simulink model "oneFingerFBSim"  (R2015b)
settings: Solver=VariableStepAuto  StartTime=0.0  StopTime=1  RelTol=1e-3
settings Model: Creator=Ricardo  LastModifiedBy=Ricardo

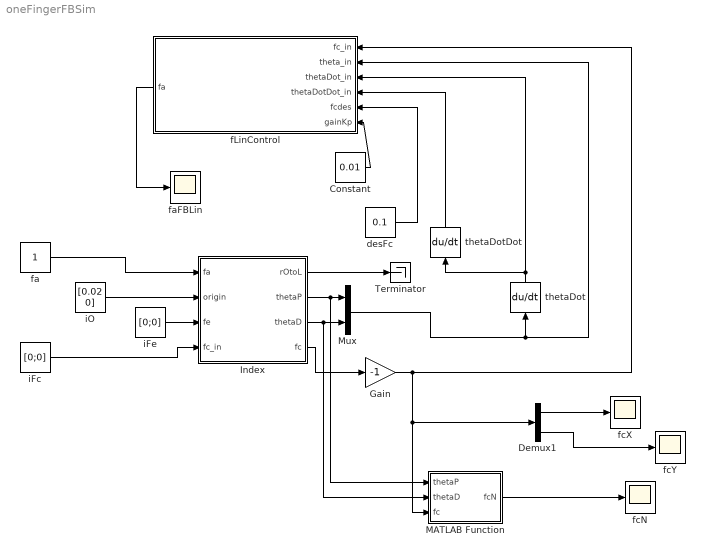
== system oneFingerFBSim ==
  Constant : Constant  Value=0.01
  Demux1 : Demux  Outputs=2
  Gain : Gain  Gain=-1
  Index : Subsystem
  MATLAB Function : MATLAB Function  TreatAsAtomicUnit=on
  Mux : Mux  Inputs=2
  Terminator : Terminator
  desFc : Constant  Value=0.1
  fLinControl : MATLAB Function  TreatAsAtomicUnit=on
  fa : Constant
  faFBLin : Scope
  fcN : Scope
  fcX : Scope
  fcY : Scope
  iFc : Constant  Value=[0;0]
  iFe : Constant  Value=[0;0]
  iO : Constant  Value=[0.02 0]
  thetaDot : Derivative
  thetaDotDot : Derivative
  wires:
  Demux1/1 -> fcX/1
  Demux1/2 -> fcY/1
  iO/1 -> Index/2(origin)
  Index/4(fc) -> Gain/1
  Index/2(thetaP) -> MATLAB Function/1(thetaP), Mux/1
  Index/3(thetaD) -> MATLAB Function/2(thetaD), Mux/2
  Mux/1 -> thetaDot/1, fLinControl/2(theta_in)
  desFc/1 -> fLinControl/5(fcdes)
  fLinControl/1(fa) -> faFBLin/1
  thetaDot/1 -> thetaDotDot/1, fLinControl/3(thetaDot_in)
  thetaDotDot/1 -> fLinControl/4(thetaDotDot_in)
  Constant/1 -> fLinControl/6(gainKp)
  iFe/1 -> Index/3(fe)
  Gain/1 -> MATLAB Function/3(fc), Demux1/1, fLinControl/1(fc_in)
  Index/1(rOtoL) -> Terminator/1
  MATLAB Function/1(fcN) -> fcN/1
  fa/1 -> Index/1(fa)
  iFc/1 -> Index/4(fc_in)

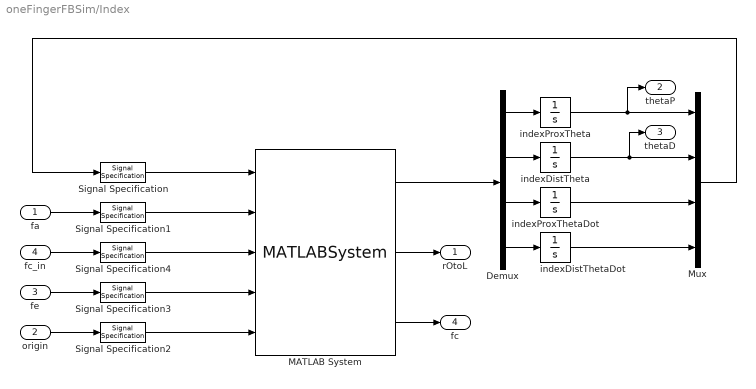
== system oneFingerFBSim/Index ==
  fa : Inport
  origin : Inport  Port=2
  fe : Inport  Port=3
  fc_in : Inport  Port=4
  Demux : Demux
  MATLAB System : MATLABSystem  System=Index  kP=-0.043  kD=-0.185  dP=-0.01  dD=-0.01  lP=0.1  lD=0.1  rP=0.02  rD=0.012  mP=0.02  mD=0.02  thetaP=pi/10  thetaD=pi/3  SimulateUsing=Interpreted execution
      mask Type: Index
      mask Display:
      | disp('Index');
      | port_label('input',1,'initVal');
      | port_label('input',2,'fa');
      | port_label('input',3,'fc');
      | port_label('input',4,'fe');
      | port_label('input',5,'origin');
      | port_label('output',1,'xDot');
      | port_label('output',2,'rOtoL');
      | port_label('output',3,'fc');
  Mux : Mux
  Signal Specification : SignalSpecification  Dimensions=4
  Signal Specification1 : SignalSpecification  Dimensions=1
  Signal Specification2 : SignalSpecification  Dimensions=2
  Signal Specification3 : SignalSpecification  Dimensions=2
  Signal Specification4 : SignalSpecification  Dimensions=2
  indexDistTheta : Integrator  InitialCondition=pi/3  ContinuousStateAttributes='indexDistTheta'
  indexDistThetaDot : Integrator  ContinuousStateAttributes='indexDistThetaDot'
  indexProxTheta : Integrator  InitialCondition=pi/10  ContinuousStateAttributes='indexProxTheta'
  indexProxThetaDot : Integrator  ContinuousStateAttributes='indexProxThetaDot'
  rOtoL : Outport
  thetaP : Outport  Port=2
  thetaD : Outport  Port=3
  fc : Outport  Port=4
  wires:
  Demux/1 -> indexProxTheta/1
  Demux/2 -> indexDistTheta/1
  Demux/3 -> indexProxThetaDot/1
  Demux/4 -> indexDistThetaDot/1
  MATLAB System/1 -> Demux/1
  indexProxTheta/1 -> Mux/1, thetaP/1
  indexDistTheta/1 -> Mux/2, thetaD/1
  indexProxThetaDot/1 -> Mux/3
  indexDistThetaDot/1 -> Mux/4
  Mux/1 -> Signal Specification/1
  Signal Specification/1 -> MATLAB System/1
  MATLAB System/2 -> rOtoL/1
  MATLAB System/3 -> fc/1
  Signal Specification1/1 -> MATLAB System/2
  fa/1 -> Signal Specification1/1
  origin/1 -> Signal Specification2/1
  Signal Specification2/1 -> MATLAB System/5
  fe/1 -> Signal Specification3/1
  Signal Specification3/1 -> MATLAB System/4
  fc_in/1 -> Signal Specification4/1
  Signal Specification4/1 -> MATLAB System/3

== matlab function oneFingerFBSim/MATLAB Function ==
  data: thetaP input; fcN output; thetaD input; fc input
function fcN = transFc(thetaP,thetaD,fc)
%#codegen

fcTN = [[cos(thetaP+thetaD),sin(thetaP+thetaD)];[-sin(thetaP+thetaD),cos(thetaP+thetaD)]]*fc;
fcN=fcTN(2,1);

== matlab function oneFingerFBSim/fLinControl ==
  data: fc_in input; theta_in input; fa output; thetaDot_in input; thetaDotDot_in input; fcdes input; gainKp input
function fa = fLinControl(fc_in,theta_in,thetaDot_in,thetaDotDot_in,fcdes,gainKp)
    theta = [theta_in(1);theta_in(2)];
    thetaDot = [thetaDot_in(1);thetaDot_in(2)];
    thetaDotDot = [thetaDotDot_in(1);thetaDotDot_in(2)];
	% Set model variables:
    kP = -0.043;
    kD = -0.185;
    dP = -0.01;
    dD = -0.01;
    lP = 0.1;
    lD = 0.1;
    rP = 0.02;
    rD = 0.012;
    aP = 0.1;
    aD = 0.1;
    mP = 0.02;
    mD = 0.02;
    theta0 = [pi/10;pi/3];
    IP = mP*(lP^2)/3;
    ID = mD*(lD^2)/12;
    % Set matrices
    K = [kP 0;
         0 kD];
    D = [dP 0;
         0 dD];
    Ja = [rP rD];
    Jc = [aP, 0;
          aD+lP*cos(theta(2,1)),aD]; 
    % Compute matrix parameters.
    alpha = IP + ID + (mP*(lP/2)^2) + mD*(lP^2+(lD/2)^2);
    beta = mD*lP*(lD/2);
    delta = ID+mD*(lD/2)^2;
    % Intertia matrix (M)
    M = [alpha+2*beta*cos(theta(2,1)) delta+beta*cos(theta(2,1));
         delta+beta*cos(theta(2,1)) delta];
    % Coriolis and Centrifugal matrix (C)
    C = [-beta*sin(theta(2,1))*thetaDot(2,1) ...
         -beta*sin(theta(2,1))*(thetaDot(1,1)+thetaDot(2,1));
         beta*sin(theta(2,1))*thetaDot(1,1) 0];
    springTau = K*(theta-theta0);
    damperTau = D*thetaDot;
    % Contact force
    fc = rotMat(theta(1,1)+theta(2,1))'*fc_in;
    fcN = fc(2,1);
    e = [0;fcdes-fcN];
    fa = pinv(Ja')*(M*thetaDotDot+C*thetaDot-springTau-damperTau-Jc'*([0;fcN]-gainKp*e));
end
        function rot = rotMat(theta)
            % 2D Z-Rotation matrix on theta.
            % @param theta the angle
            % @return rot the rotation matrix as a 2x2 matrix.
            rot = [cos(theta) -sin(theta);
                   sin(theta) cos(theta)];
        end
